simulink model "mbqpsk"  (R2019a)
settings: Solver=FixedStepDiscrete  StartTime=0.0  StopTime=inf  RelTol=1e-3  EnableMultiTasking=on
PreLoadFcn:
  | SimPars = simrfV2_qpsk_init();
  | load simrfV2_qpsk_patch_antenna.mat;
undefined symbols (not defined in the file or in its folder): lambda, P_isolated, phased, physconst
libraries: simrfV2util1 x44, simrfV2elements x40, simrfV2junction1 x28, simrfV2systems x8, commrflib2 x3, commdigbbndpm3 x3, dspsigops x3, dspmathops x3, phasedtxrxlib x3, commutil2 x2, commsequence2 x2, commsync2 x2
(part 1 of 2)
CloseFcn:
  | clear SimPars lambda P_isolated;
  | clear Spars;
Description:
  | Modeling an RF mmWave Transmitter with Hybrid Beamforming
settings Model: SimulationMode=accelerator  Creator=Arpan Samanta  LastModifiedBy=Arpan
settings DataIOCC: ExternalInput=txWaveform  InitialState=xFinal  SaveOperatingPoint=on  SaveFormat=Array  SaveOutput=off  SignalLogging=off  DSMLogging=off  SaveTime=off  ReturnWorkspaceOutputs=off  OutputSaveName=rx
settings OptimizationCC: DefaultParameterBehavior=Inlined  InlineInvariantSignals=on  EfficientMapNaN2IntZero=off  LifeSpan=inf  SimCompilerOptimization=on
settings DebuggingCC: ReadBeforeWriteMsg=DisableAll  WriteAfterWriteMsg=DisableAll  WriteAfterReadMsg=DisableAll  UnderspecifiedInitializationDetection=Classic  MergeDetectMultiDrivingBlocksExec=none  SolverPrmCheckMsg=warning  InheritedTsInSrcMsg=none  MultiTaskDSMMsg=none  IntegerOverflowMsg=none  AllowSymbolicDim=off  SFUnexpectedBacktrackingDiag=warning  SFNoUnconditionalDefaultTransitionDiag=none  SFUndirectedBroadcastEventsDiag=none  SFExecutionAtInitializationDiag=none  IntegerSaturationMsg=none  ArithmeticOperatorsInVariantConditions=warning
settings HardwareCC: ProdBitPerPointer=32  ProdBitPerSizeT=32  ProdBitPerPtrDiffT=32  ProdLargestAtomicFloat=None  ProdIntDivRoundTo=Undefined  ProdEndianess=Unspecified  ProdWordSize=32  ProdHWDeviceType=32-bit Generic  TargetBitPerPointer=64  TargetBitPerSizeT=64  TargetBitPerPtrDiffT=64  TargetLongLongMode=on  TargetIntDivRoundTo=Zero  TargetEndianess=LittleEndian  TargetWordSize=64  TargetHWDeviceType=MATLAB Host  ProdEqTarget=off
settings ModelReferenceCC: EnableParallelModelReferenceBuilds=on  PropagateSignalLabelsOutOfModel=off
settings SFSimCC: SFSimEcho=off  SimUseLocalCustomCode=off
settings RTWCC: RTWUseLocalCustomCode=off  BuildConfiguration=Faster Runs
settings CodeAppCC: MaxIdLength=128  StateflowObjectComments=on
settings GRTTargetCC: TargetLangStandard=C89/C90 (ANSI)  CombineOutputUpdateFcns=off  GRTInterface=on
settings ConfigComp: CovMetricSettings=dw  CovHtmlReporting=on  CovSaveCumulativeToWorkspaceVar=on  CovSaveSingleToWorkspaceVar=on  CovExternalEMLEnable=off  CovSFcnEnable=off
settings SimscapeCC: ExplicitSolverDiagnosticOptions=none  SimscapeNormalizeSystem=off

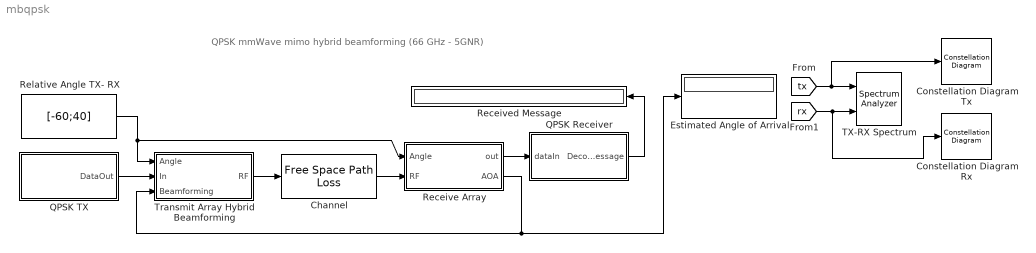
== system mbqpsk ==
  note: QPSK mmWave mimo hybrid beamforming (66 GHz - 5GNR)
  Channel : commrflib2/Free Space Path Loss  mode=Decibels  dB=50  d=0.100  fc=1920
      settings: SourceProductName=Communications Toolbox  SourceProductBaseCode=CM
  Constellation Diagram Rx : ConstellationDiagram
  Constellation Diagram Tx : ConstellationDiagram
  Estimated Angle of Arrival : Display
  QPSK Receiver : Subsystem
      mask Display: disp('QPSK \n Receiver');
  QPSK TX : Subsystem  mask{Power=-30}
      mask prompts: Power "Power (dBFS)"
      mask Display: disp('QPSK \n Transmitter')
  Receive Array : Subsystem
  Received Message : Display
  Relative Angle TX- RX : Constant  Value=[-60;40]  VectorParams1D=off
  TX-RX Spectrum : SpectrumAnalyzer  NumInputPorts=2
  Transmit Array Hybrid Beamforming : Subsystem
  wires:
  Channel/1 -> Receive Array/2(RF)
  Receive Array/1(out) -> QPSK Receiver/1(dataIn)
  Relative Angle TX- RX/1 -> Transmit Array Hybrid Beamforming/1(Angle), Receive Array/1(Angle)
  [tx] -> TX-RX Spectrum/1, Constellation Diagram Tx/1
  [rx] -> TX-RX Spectrum/2, Constellation Diagram Rx/1
  QPSK Receiver/1(Decoded Message) -> Received Message/1
  QPSK TX/1(DataOut) -> Transmit Array Hybrid Beamforming/2(In)
  Transmit Array Hybrid Beamforming/1(RF) -> Channel/1
  Receive Array/2(AOA) -> Estimated Angle of Arrival/1, Transmit Array Hybrid Beamforming/3(Beamforming)

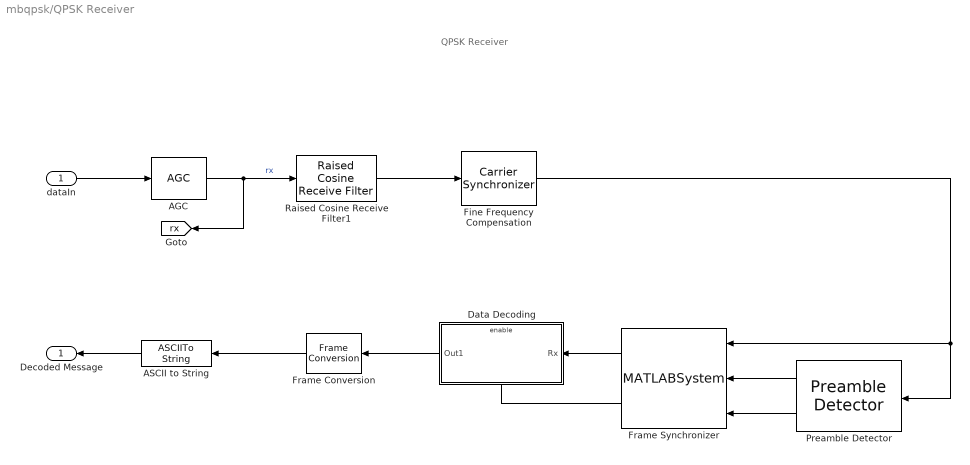
== system mbqpsk/QPSK Receiver ==
  note: QPSK Receiver
  dataIn : Inport
  AGC : commrfcorlib/AGC  LegacyMode=off  DetectorMethod=Rectifier  LoopMethod=Linear  UpdatePeriod=100  StepSize=0.1  AdaptationStepSize=0.01  DesiredOutputPower=1  AveragingLength=200  MaximumGain=30  MaxPowerGain=60  GainOutputPort=off  InputPowerOutputPort=off  SimulateUsing=Code generation
      settings: SourceProductName=Communications Toolbox
  ASCII to String : ASCIIToString
  Data Decoding : Subsystem
      mask Display: disp('Data Decoding');
  Fine Frequency Compensation : commsync2/Carrier Synchronizer  Modulation=QPSK  ModulationPhaseOffset=Auto  CustomPhaseOffset=0  SamplesPerSymbol=1  DampingFactor=1/sqrt(2)  NormalizedLoopBandwidth=0.005  EstimatedPhaseErrorOutputPort=off  SimulateUsing=Code generation
      settings: SourceProductName=Communications Toolbox
  Frame Conversion : FrameConversion  OutFrame=Sample-based
  Frame Synchronizer : MATLABSystem  System=comm.internal.examples.FrameSynchronizer  Input=Symbol  OutputFrameLength=SimPars.NumSymsPerFrame  PreambleLength=SimPars.BarkerLength  SimulateUsing=Code generation
      mask Type: comm.internal.examples.FrameSynchronizer
      mask Display:
      | disp(['Frame' char(10) 'Synchronizer']);
      | port_label('input',1,'u');
      | port_label('input',2,'idx');
      | port_label('input',3,'dtMt');
      | port_label('output',1,'Frame');
      | port_label('output',2,'Valid');
  Preamble Detector : commsync2/Preamble Detector  Input=Symbol  Preamble=sqrt(2)/2 * (-1-1i) *SimPars.BarkerCode  Threshold=10  DetectionMetricOutput=on  Detections=All  SimulateUsing=Code generation
      settings: SourceProductName=Communications Toolbox  SourceProductBaseCode=CM
  Raised Cosine Receive Filter1 : commfilt2/Raised Cosine Receive Filter  filtType=Square root  R=SimPars.RolloffFactor  filtSpan=SimPars.RCFilterSpan  N=SimPars.SamplesPerSymbol  downFactor=SimPars.RxRCFilterDecimation  downOffset=0  filterGain=1  InputProcessing=Columns as channels (frame based)  RateOptions=Enforce single-rate processing  framing=Mute  checkCoeff=off  variableName=rcRxFilt1  currentFiltSpan=10  D=5  inputOffset=0  sampMode=Mute  saveAsFlag=0  rateMode=Downsampling  checkGain=Normalized  launchFVT=on  roundingMode=Floor  overflowMode=off  coeffDataTypeStr=Inherit: Same word length as input  coeffMin=[]  coeffMax=[]  coeffLastDataTypeStr=Inherit: Same word length as input  accumDataTypeStr=Inherit: Same as product output  accumLastDataTypeStr=Inherit: Same as product output  outputDataTypeStr=Inherit: Same as accumulator  outputMin=[]  outputMax=[]  outputLastDataTypeStr=Inherit: Same as accumulator
      settings: SourceProductName=Communications Toolbox
  Decoded Message : Outport
  tag scope: rx=global
  wires:
  ASCII to String/1 -> Decoded Message/1
  Frame Conversion/1 -> ASCII to String/1
  AGC/1 -> Raised Cosine Receive Filter1/1, [rx]  "rx"
  Preamble Detector/1 -> Frame Synchronizer/2
  Frame Synchronizer/2 -> Data Decoding/Enable
  Frame Synchronizer/1 -> Data Decoding/1(Rx)
  Preamble Detector/2 -> Frame Synchronizer/3
  Fine Frequency Compensation/1 -> Frame Synchronizer/1, Preamble Detector/1
  Data Decoding/1(Out1) -> Frame Conversion/1
  dataIn/1 -> AGC/1
  Raised Cosine Receive Filter1/1 -> Fine Frequency Compensation/1

== system mbqpsk/QPSK TX ==
  note: QPSK Transmitter
  Bit Generation : Subsystem
      mask Display: disp('Bits Generation')
  Gain : Gain  Gain=sqrt(2)
  QPSK Modulator Baseband : commdigbbndpm3/QPSK Modulator Baseband  InType=Bit  Enc=Gray  Ph=pi/4  outDtype=double  outWordLen=16  outUDDataType=sfix(16)  outFracLenMode=Best precision  outFracLen=15  outDataTypeStr=double  outLastDataTypeStr=double
      settings: SourceProductName=Communications Toolbox
  Raised Cosine Transmit Filter1 : commfilt2/Raised Cosine Transmit Filter  filtType=Square root  R=SimPars.RolloffFactor  filtSpan=SimPars.RCFilterSpan  N=SimPars.SamplesPerSymbol  filterGain=1  InputProcessing=Columns as channels (frame based)  RateOptions=Enforce single-rate processing  framing=Mute  checkCoeff=off  variableName=rcTxFilt1  checkGain=Normalized  sampMode=Mute  saveAsFlag=0  currentFiltSpan=10  D=5  launchFVT=on  roundingMode=Floor  overflowMode=off  coeffDataTypeStr=Inherit: Same word length as input  coeffMin=[]  coeffMax=[]  coeffLastDataTypeStr=Inherit: Same word length as input  outputDataTypeStr=Inherit: Same as accumulator  outputMin=[]  outputMax=[]  outputLastDataTypeStr=Inherit: Same as accumulator
      settings: SourceProductName=Communications Toolbox
  Unbuffer : Unbuffer
  dB Gain : dspmathops/dB Gain  dB=Power-30+3  intype=Amplitude
      settings: SourceProductName=DSP System Toolbox  SourceProductBaseCode=DS
  DataOut : Outport
  tag scope: tx=global
  wires:
  Unbuffer/1 -> DataOut/1
  dB Gain/1 -> Unbuffer/1
  Bit Generation/1(Out) -> QPSK Modulator Baseband/1
  QPSK Modulator Baseband/1 -> Raised Cosine Transmit Filter1/1
  Raised Cosine Transmit Filter1/1 -> Gain/1, dB Gain/1
  Gain/1 -> [tx]  "tx"

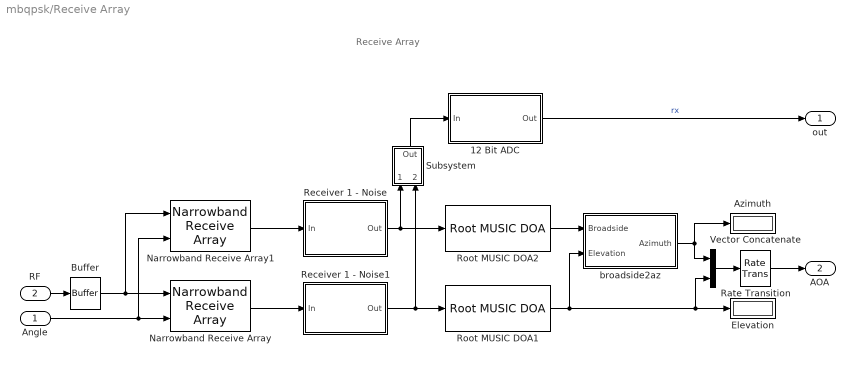
== system mbqpsk/Receive Array ==
  note: Receive Array
  Angle : Inport
  RF : Inport  Port=2
  12 Bit ADC : Subsystem  mask{FS_P_dBm=-10, N=12}
      mask prompts: FS_P_dBm "Full Scale Power (dBm)"
  Azimuth : Display
  Buffer : Buffer  N=SimPars.NumBitsPerFrame  OutputFrames=off
  Elevation : Display
  Narrowband Receive Array : phasedtxrxlib/Narrowband Receive Array  PropagationSpeed=physconst( 'LightSpeed' )  OperatingFrequency=SimPars.CarrierFreq  Wavefront=Plane  SensorGainMeasure=dB  Polarization=None  WeightsInputPort=off  SimulateUsing=Code generation  Sensor=phased.ULA('NumElements',4,'ElementSpacing',lambda/2,'ArrayAxis','z','Element',phased.IsotropicAntennaElement('BackBaffled',true))
      settings: SourceProductName=Phased Array System Toolbox  SourceProductBaseCode=AR
  Narrowband Receive Array1 : phasedtxrxlib/Narrowband Receive Array  PropagationSpeed=physconst( 'LightSpeed' )  OperatingFrequency=SimPars.CarrierFreq  Wavefront=Plane  SensorGainMeasure=dB  Polarization=None  WeightsInputPort=off  SimulateUsing=Code generation  Sensor=phased.ULA('NumElements',4,'ElementSpacing',lambda/2,'ArrayAxis','y','Element',phased.IsotropicAntennaElement('BackBaffled',true))
      settings: SourceProductName=Phased Array System Toolbox  SourceProductBaseCode=AR
  Rate Transition : RateTransition
  Receiver 1 - Noise : Subsystem  mask{NF=5, Gain=40, seed=123}
      mask prompts: NF "Noise Figure (dB)"; Gain "Gain (dB)"
      mask Display: disp('Receiver\n Gain/Noise')
  Receiver 1 - Noise1 : Subsystem  mask{NF=5, Gain=40, seed=3456}
      mask prompts: NF "Noise Figure (dB)"; Gain "Gain (dB)"
      mask Display: disp('Receiver\n Gain/Noise')
  Root MUSIC DOA1 : phaseddoalib/Root MUSIC DOA  PropagationSpeed=physconst( 'LightSpeed' )  OperatingFrequency=SimPars.CarrierFreq  NumSignalsSource=Property  NumSignalsMethod=AIC  NumSignals=1  ForwardBackwardAveraging=off  SpatialSmoothing=0  SimulateUsing=Code generation  SensorArray=phased.ULA('Element',phased.IsotropicAntennaElement('BackBaffled',true),'NumElements',4,'ElementSpacing',lambda/2,'ArrayAxis','z')
      settings: SourceProductName=Phased Array System Toolbox  SourceProductBaseCode=AR
  Root MUSIC DOA2 : phaseddoalib/Root MUSIC DOA  PropagationSpeed=physconst( 'LightSpeed' )  OperatingFrequency=SimPars.CarrierFreq  NumSignalsSource=Property  NumSignalsMethod=AIC  NumSignals=1  ForwardBackwardAveraging=off  SpatialSmoothing=0  SimulateUsing=Code generation  SensorArray=phased.ULA('Element',phased.IsotropicAntennaElement('BackBaffled',true),'NumElements',4,'ElementSpacing',0.5*lambda)
      settings: SourceProductName=Phased Array System Toolbox  SourceProductBaseCode=AR
  Subsystem : Subsystem
  Vector Concatenate : Concatenate  Mode=Multidimensional array
  broadside2az : Subsystem  VariantControl=BroadsideToAzimuth
  out : Outport
  AOA : Outport  Port=2
  wires:
  RF/1 -> Buffer/1
  broadside2az/1(Azimuth) -> Azimuth/1, Vector Concatenate/1
  Vector Concatenate/1 -> Rate Transition/1
  Angle/1 -> Narrowband Receive Array1/2, Narrowband Receive Array/2
  Root MUSIC DOA2/1 -> broadside2az/1(Broadside)
  Root MUSIC DOA1/1 -> Elevation/1, Vector Concatenate/2, broadside2az/2(Elevation)
  Narrowband Receive Array/1 -> Receiver 1 - Noise1/1(In)
  Narrowband Receive Array1/1 -> Receiver 1 - Noise/1(In)
  Receiver 1 - Noise/1(Out) -> Root MUSIC DOA2/1, Subsystem/1(In1)
  Receiver 1 - Noise1/1(Out) -> Root MUSIC DOA1/1, Subsystem/2(In2)
  Buffer/1 -> Narrowband Receive Array1/1, Narrowband Receive Array/1
  Rate Transition/1 -> AOA/1
  12 Bit ADC/1(Out) -> out/1  "rx"
  Subsystem/1(Out) -> 12 Bit ADC/1("In  ")

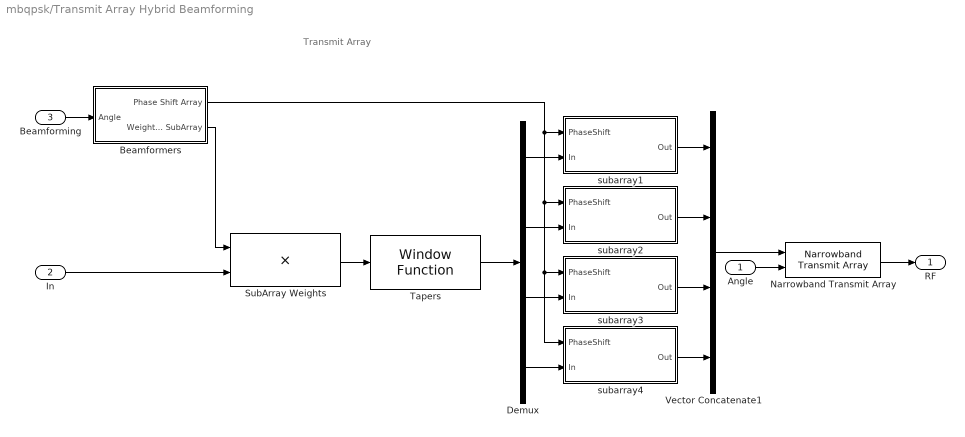
== system mbqpsk/Transmit Array Hybrid Beamforming ==
  note: Transmit Array
  Angle : Inport
  In : Inport  Port=2
  Beamforming : Inport  Port=3
  Beamformers : Subsystem
  Demux : Demux
  Narrowband Transmit Array : phasedtxrxlib/Narrowband Transmit Array  PropagationSpeed=physconst( 'LightSpeed' )  OperatingFrequency=SimPars.CarrierFreq  CombineRadiatedSignals=on  SensorGainMeasure=dB  Polarization=None  WeightsInputPort=off  SimulateUsing=Interpreted execution  Sensor=phased.URA('Size',[8, 4],'ElementSpacing',[0.5*lambda, 0.5*lambda],'Element',phased.CustomAntennaElement('AzimuthAngles',-180:5:180,'ElevationAngles',-90:5:90,'MagnitudePattern',P_isolated,'PhasePattern',zeros(37,73)))
      settings: SourceProductName=Phased Array System Toolbox  SourceProductBaseCode=AR
  SubArray Weights : Product
  Tapers : dspsigops/Window Function  winmode=Apply window to input  wintype=Hamming  sampmode=Continuous  samptime=1  N=64  Rs=50  beta=10  winsamp=Symmetric  UserWindow=hamming  OptParams=off  UserParams={'symmetric'}  dataType=double  isSigned=on  wordLen=16  udDataType=sfix(16)  fracBitsMode=Best precision  numFracBits=15  roundingMode=Floor  overflowMode=off  numSidelobes=4  sidelobeLevel=-30
      settings: SourceProductName=DSP System Toolbox  SourceProductBaseCode=DS
  Vector Concatenate1 : Concatenate  NumInputs=4  Mode=Multidimensional array  ConcatenateDimension=2
  subarray1 : Subsystem
  subarray2 : Subsystem
  subarray3 : Subsystem
  subarray4 : Subsystem
  RF : Outport
  wires:
  Demux/1 -> subarray1/2(In)
  Demux/2 -> subarray2/2(In)
  Demux/3 -> subarray3/2(In)
  Demux/4 -> subarray4/2(In)
  subarray1/1(Out) -> Vector Concatenate1/1
  subarray2/1(Out) -> Vector Concatenate1/2
  subarray3/1(Out) -> Vector Concatenate1/3
  subarray4/1(Out) -> Vector Concatenate1/4
  SubArray Weights/1 -> Tapers/1
  Beamformers/1(Phase Shift Array) -> subarray1/1(PhaseShift), subarray2/1(PhaseShift), subarray3/1(PhaseShift), subarray4/1(PhaseShift)
  Narrowband Transmit Array/1 -> RF/1
  Beamformers/2(Weights SubArray) -> SubArray Weights/1
  Beamforming/1 -> Beamformers/1(Angle)
  Vector Concatenate1/1 -> Narrowband Transmit Array/1
  In/1 -> SubArray Weights/2
  Angle/1 -> Narrowband Transmit Array/2
  Tapers/1 -> Demux/1

== system mbqpsk/QPSK Receiver/Data Decoding ==
  Rx : Inport
  Enable : EnablePort
  "Barker Code Symbol Generation " : Subsystem
      mask Display: disp('Barker Code\nSymbol Generation')
  Bit to Integer Converter : commutil2/Bit to Integer Converter  nbits=7  bitOrder=MSB first  signedOutputValues=Unsigned  outDtype=Inherit via internal rule  outDtypeSigned=Inherit via internal rule
      settings: SourceProductName=Communications Toolbox
  Descrambling : Subsystem
      mask Display: disp('Descrambling');
  Phase Ambiguity Correction & Demodulation : Subsystem
      mask Display: disp('Phase Ambiguity\nCorrection\n& Demodulation');
  Phase Offset Estimator : Subsystem
  Out1 : Outport
  wires:
  "Barker Code Symbol Generation "/1(Out) -> Phase Offset Estimator/1(BarkerRef)
  Phase Offset Estimator/1(Phase) -> Phase Ambiguity Correction & Demodulation/1(Phase)
  Rx/1 -> Phase Offset Estimator/2(Data), Phase Ambiguity Correction & Demodulation/2(Data)
  Descrambling/1(Out) -> Bit to Integer Converter/1
  Phase Ambiguity Correction & Demodulation/1(Out) -> Descrambling/1(In)
  Bit to Integer Converter/1 -> Out1/1

== system mbqpsk/QPSK TX/Bit Generation ==
  note: Each data frame contains 26 bits header (For Sync Purpose) and 174 data bits, first 105 data bits contain "Hello world ###" message. Scrambler is there to improve data transition density and frequency offset estimation.
  Barker Code SS : Subsystem
      mask Display: disp('Unipolar\nBarker Code')
  Matrix Concatenate : Concatenate  Mode=Multidimensional array
  Message Source : Subsystem
      mask Display: disp('Message\nSource')
  Repeat : dspsigops/Repeat  N=2  InputProcessing=Columns as channels (frame based)  RateOptions=Enforce single-rate processing  ic=0  mode=Unused parameter value
      settings: SourceProductName=DSP System Toolbox
  Scrambler : commsequence2/Scrambler  M=2  poly=[1 1 1 0 1]  iniStaSource=Dialog Parameter  ini_sta=[0 0 0 0]  resetViaPort=off
      settings: SourceProductName=Communications Toolbox  SourceProductBaseCode=CM
  Out : Outport
  wires:
  Barker Code SS/1(Out) -> Repeat/1
  Matrix Concatenate/1 -> Out/1
  Message Source/1(Out) -> Scrambler/1
  Repeat/1 -> Matrix Concatenate/1
  Scrambler/1 -> Matrix Concatenate/2

== system mbqpsk/Receive Array/12 Bit ADC ==
  "In  " : Inport
  Complex to Real-Imag : ComplexToRealImag
  Idealized ADC quantizer : simulink_extras/Additional Discrete/Idealized ADC quantizer  NumberOfConverterBits=N  Vmin=-10^((FS_P_dBm-30)/20)  Vmax=10^((FS_P_dBm-30)/20)  OutputDataType=double  OutputNegativeValues=on
      settings: SourceProductName=Simulink
  Idealized ADC quantizer1 : simulink_extras/Additional Discrete/Idealized ADC quantizer  NumberOfConverterBits=N  Vmin=-10^((FS_P_dBm-30)/20)  Vmax=10^((FS_P_dBm-30)/20)  OutputDataType=double  OutputNegativeValues=on
      settings: SourceProductName=Simulink
  Real-Imag to Complex : RealImagToComplex
  Out : Outport
  wires:
  "In  "/1 -> Complex to Real-Imag/1
  Complex to Real-Imag/1 -> Idealized ADC quantizer/1
  Complex to Real-Imag/2 -> Idealized ADC quantizer1/1
  Idealized ADC quantizer/1 -> Real-Imag to Complex/1
  Idealized ADC quantizer1/1 -> Real-Imag to Complex/2
  Real-Imag to Complex/1 -> Out/1

== system mbqpsk/Receive Array/Receiver 1 - Noise ==
  In : Inport
  Convert 1-D to 2-D : dspsigattribs/Convert 1-D to 2-D  M=200 % Frame  N=4  frameBasedOut=off
      settings: SourceProductName=DSP System Toolbox  SourceProductBaseCode=DS
  Receiver Thermal Noise : commrflib2/Receiver Thermal Noise  method=Noise figure  ntemp=290  nfigure=NF  nfactor=2  add290KAntennaNoise=on  seed=seed
      settings: SourceProductName=Communications Toolbox  SourceProductBaseCode=CM
  Reshape : Reshape  OutputDimensionality=Column vector (2-D)
  dB Gain : dspmathops/dB Gain  dB=Gain  intype=Amplitude
      settings: SourceProductName=DSP System Toolbox  SourceProductBaseCode=DS
  Out : Outport
  wires:
  In/1 -> Reshape/1
  Reshape/1 -> Receiver Thermal Noise/1
  Receiver Thermal Noise/1 -> dB Gain/1
  Convert 1-D to 2-D/1 -> Out/1
  dB Gain/1 -> Convert 1-D to 2-D/1

== system mbqpsk/Receive Array/Receiver 1 - Noise1 ==
  In : Inport
  Convert 1-D to 2-D : dspsigattribs/Convert 1-D to 2-D  M=200 % Frame  N=4  frameBasedOut=off
      settings: SourceProductName=DSP System Toolbox  SourceProductBaseCode=DS
  Receiver Thermal Noise : commrflib2/Receiver Thermal Noise  method=Noise figure  ntemp=290  nfigure=NF  nfactor=2  add290KAntennaNoise=on  seed=seed
      settings: SourceProductName=Communications Toolbox  SourceProductBaseCode=CM
  Reshape : Reshape  OutputDimensionality=Column vector (2-D)
  dB Gain : dspmathops/dB Gain  dB=Gain  intype=Amplitude
      settings: SourceProductName=DSP System Toolbox  SourceProductBaseCode=DS
  Out : Outport
  wires:
  dB Gain/1 -> Convert 1-D to 2-D/1
  Convert 1-D to 2-D/1 -> Out/1
  Receiver Thermal Noise/1 -> dB Gain/1
  Reshape/1 -> Receiver Thermal Noise/1
  In/1 -> Reshape/1

== system mbqpsk/Receive Array/Subsystem ==
  In1 : Inport
  In2 : Inport  Port=2
  Add : Sum
  Sum of Elements : Sum  Inputs=+  CollapseMode=Specified dimension  CollapseDim=2
  Sum of Elements1 : Sum  Inputs=+  CollapseMode=Specified dimension  CollapseDim=2
  Out : Outport
  wires:
  Sum of Elements/1 -> Add/1
  Sum of Elements1/1 -> Add/2
  Add/1 -> Out/1
  In2/1 -> Sum of Elements1/1
  In1/1 -> Sum of Elements/1

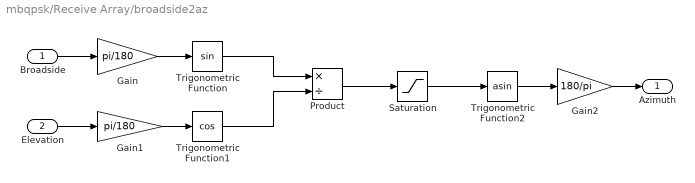
== system mbqpsk/Receive Array/broadside2az ==
  Broadside : Inport
  Elevation : Inport  Port=2
  Gain : Gain  Gain=pi/180
  Gain1 : Gain  Gain=pi/180
  Gain2 : Gain  Gain=180/pi
  Product : Product  Inputs=*/
  Saturation : Saturate  UpperLimit=1  LowerLimit=-1
  Trigonometric Function : Trigonometry
  Trigonometric Function1 : Trigonometry  Operator=cos
  Trigonometric Function2 : Trigonometry  Operator=asin
  Azimuth : Outport
  wires:
  Product/1 -> Saturation/1
  Gain2/1 -> Azimuth/1
  Trigonometric Function1/1 -> Product/2
  Trigonometric Function/1 -> Product/1
  Trigonometric Function2/1 -> Gain2/1
  Gain/1 -> Trigonometric Function/1
  Broadside/1 -> Gain/1
  Elevation/1 -> Gain1/1
  Gain1/1 -> Trigonometric Function1/1
  Saturation/1 -> Trigonometric Function2/1

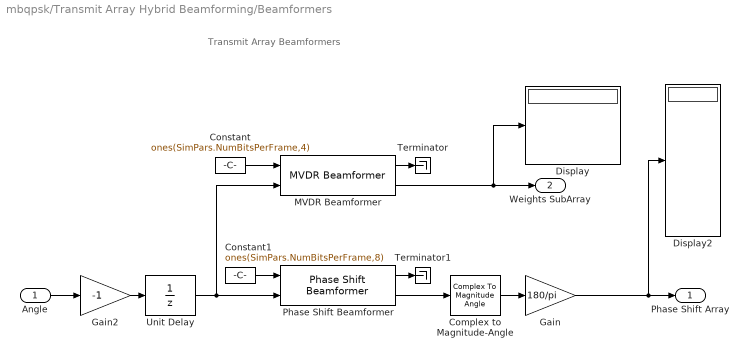
== system mbqpsk/Transmit Array Hybrid Beamforming/Beamformers ==
  note: Transmit Array Beamformers
  Angle : Inport
  Complex to Magnitude-Angle : ComplexToMagnitudeAngle  Output=Angle
  Constant : Constant  Value=ones(SimPars.NumBitsPerFrame,4)  VectorParams1D=off
  Constant1 : Constant  Value=ones(SimPars.NumBitsPerFrame,8)  VectorParams1D=off
  Display : Display
  Display2 : Display
  Gain : Gain  Gain=180/pi
  Gain2 : Gain  Gain=-1
  MVDR Beamformer : phasedbflib/MVDR Beamformer  PropagationSpeed=physconst( 'LightSpeed' )  OperatingFrequency=SimPars.CarrierFreq  DiagonalLoadingFactor=0.1  TrainingInputPort=off  DirectionSource=Input port  Direction=[ 0; 0 ]  NumPhaseShifterBits=0  WeightsOutputPort=on  SimulateUsing=Interpreted execution  SensorArray=phased.ReplicatedSubarray('GridSize',[ 1, 4],'GridSpacing',lambda/2,'SubarraySteering','Phase','PhaseShifterFrequency',SimPars.CarrierFreq,'Subarray',phased.ULA('NumElements',8,'ElementSpacing',lambda,'ArrayAxis','z','Element',phased.CustomAntennaElement('AzimuthAngles',-180:5:180,'ElevationAngles',-90:5:90,'MagnitudePattern',P_isolated,'PhasePattern',zeros(37,73))))
      settings: SourceProductName=Phased Array System Toolbox  SourceProductBaseCode=AR
  Phase Shift Beamformer : phasedbflib/Phase Shift Beamformer  PropagationSpeed=physconst( 'LightSpeed' )  OperatingFrequency=SimPars.CarrierFreq  DirectionSource=Input port  Direction=[ 0; 0 ]  NumPhaseShifterBits=0  WeightsNormalization=Distortionless  WeightsOutputPort=on  SimulateUsing=Interpreted execution  SensorArray=phased.ULA('Element',phased.CustomAntennaElement('AzimuthAngles',-180:5:180,'ElevationAngles',-90:5:90,'MagnitudePattern',P_isolated,'PhasePattern',zeros(37,73)),'NumElements',8,'ElementSpacing',0.5*lambda,'ArrayAxis','z')
      settings: SourceProductName=Phased Array System Toolbox  SourceProductBaseCode=AR
  Terminator : Terminator
  Terminator1 : Terminator
  Unit Delay : UnitDelay  SampleTime=-1  HasFrameUpgradeWarning=on
  Phase Shift Array : Outport
  Weights SubArray : Outport  Port=2
  wires:
  MVDR Beamformer/1 -> Terminator/1
  Complex to Magnitude-Angle/1 -> Gain/1
  Constant1/1 -> Phase Shift Beamformer/1
  Angle/1 -> Gain2/1
  Phase Shift Beamformer/1 -> Terminator1/1
  Constant/1 -> MVDR Beamformer/1
  Gain/1 -> Phase Shift Array/1, Display2/1
  Gain2/1 -> Unit Delay/1
  Unit Delay/1 -> MVDR Beamformer/2, Phase Shift Beamformer/2
  MVDR Beamformer/2 -> Weights SubArray/1, Display/1
  Phase Shift Beamformer/2 -> Complex to Magnitude-Angle/1

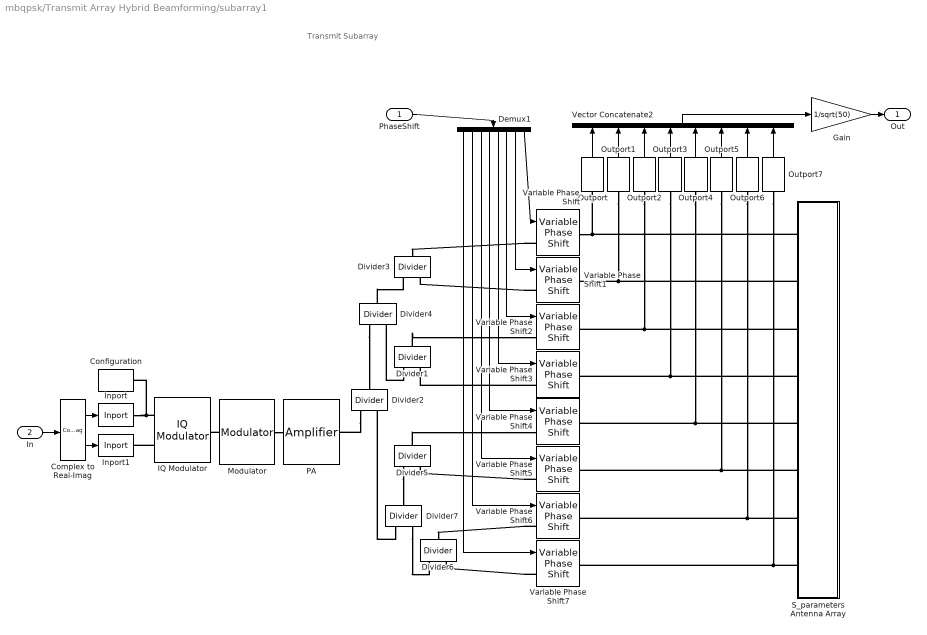
== system mbqpsk/Transmit Array Hybrid Beamforming/subarray1 ==
  note: Transmit Subarray
  PhaseShift : Inport  OutDataTypeStr=double  PortDimensions=[8 1]  SampleTime=[1.3020833333333334e-07,0]
  In : Inport  Port=2  OutDataTypeStr=double  PortDimensions=[1 1]  SampleTime=[1.3020833333333334e-07,0]
      settings: SignalType=complex
  Complex to Real-Imag : ComplexToRealImag
  Configuration : simrfV2util1/Configuration  AutoFreq=off  Tones="[5  66] GHz"  Harmonics=[3 1]  NormalizeCarrierPower=on  SolverType=Auto  UseCCode=on  StepSize=SimPars.SampleTime s  AddNoise=on  defaultRNG=on  Seed=0  Temperature=290.0 K  SolverDelFlag=0  AbsTol=1e-6  RelTol=1e-3  MaxIter=10  ErrorEstimationType=2-norm over all variables  EnableInterpFilter=off  HiddenFIRfilterControllerParam=off  SmallSignalApprox=off  AllSimFreqs=on  SimFreqs=[] Hz  SimFreqsInternal=[]
      settings: SourceProductName=RF Blockset  SourceProductBaseCode=RB
  Demux1 : Demux  Outputs=8
  Divider{1..7} (7 alike) : simrfV2junction1/Divider  classname=dividers  DataSource=Network-parameters  NumPorts=3  DeviceCirculator=Circulator clockwise  DeviceDivider=Wilkinson power divider  DeviceCoupler=Directional coupler  Paramtype=S-parameters  Sparam=[0 0 1; 1 0 0; 0 1 0]  SparamFreq=1e9 Hz  SparamZ0=50  Phase12=0  Phase33=0  Alpha=0  Coupling=0  Directivity=inf  InsertionLoss=inf  ReturnLoss=inf  InternalGrounding=on  SparamRepresentation=Frequency domain  FitOpt=Share all poles  FitTol=-40
      settings: SourceProductName=RF Blockset  SourceProductBaseCode=RB
  Gain : Gain  Gain=1/sqrt(50)
  IQ Modulator : simrfV2systems/IQ Modulator  classname=iqmod  Source_linear_gain=Available power gain  linear_gain=8 dB  Poly_Coeffs=[0 1]  LOFreq=5e9 Hz  Zin=50  Zout=50  AddIRFilters=off  AddCSFilter=off  InternalGrounding=on  ForceNextInit=off  NFloor=-168  GainMismatch=0.1 dB  PhaseMismatch=1.2 deg  Isolation=80 dB  AddPhaseNoise=off  PhaseNoiseOffset=1  PhaseNoiseLevel=-Inf  AutoImpulseLengthPN=on  ImpulseLengthPN=1e-10  ImpulseLength_unitPN=s  Source_Poly=Even and odd order  IPType=Output  IP2=21 dBm  IP3=30 dBm  P1dB=inf dBm  Psat=inf dBm  Gcomp=inf dBm  DesignMethodIR=Ideal  ResponseTypeIR=Lowpass  ImplementationIR=LC Tee  ImplementationIdealIR=Constant per carrier  UseFilterOrderIR=on  FilterOrderIR=3  PassFreq_lpIR=1  PassFreq_lp_unitIR=GHz  PassFreq_hpIR=2  PassFreq_hp_unitIR=GHz  PassFreq_bpIR=[2 3]  PassFreq_bp_unitIR=GHz  PassFreq_bsIR=[1 4]  PassFreq_bs_unitIR=GHz  PassAttenIR=10*log10(2)  StopFreq_lpIR=2  StopFreq_lp_unitIR=GHz  StopFreq_hpIR=1  StopFreq_hp_unitIR=GHz  StopFreq_bpIR=[1.5 3.5]  StopFreq_bp_unitIR=GHz  StopFreq_bsIR=[2.1 2.9]  StopFreq_bs_unitIR=GHz  StopAttenIR=40  RsrcIR=50  RloadIR=50  AutoImpulseLengthIR=on  ImpulseLengthIR=1e-10  ImpulseLength_unitIR=s  DesignMethodCS=Ideal  ResponseTypeCS=Highpass  ImplementationCS=LC Tee  ImplementationIdealCS=Constant per carrier  UseFilterOrderCS=on  FilterOrderCS=3  PassFreq_lpCS=1  PassFreq_lp_unitCS=GHz  PassFreq_hpCS=2  PassFreq_hp_unitCS=GHz  PassFreq_bpCS=[2 3]  PassFreq_bp_unitCS=GHz  PassFreq_bsCS=[1 4]  PassFreq_bs_unitCS=GHz  PassAttenCS=10*log10(2)  StopFreq_lpCS=2  StopFreq_lp_unitCS=GHz  StopFreq_hpCS=1  StopFreq_hp_unitCS=GHz  StopFreq_bpCS=[1.5 3.5]  StopFreq_bp_unitCS=GHz  StopFreq_bsCS=[2.1 2.9]  StopFreq_bs_unitCS=GHz  StopAttenCS=40  RsrcCS=50  RloadCS=50  AutoImpulseLengthCS=on  ImpulseLengthCS=1e-10  ImpulseLength_unitCS=s
      settings: SourceProductName=RF Blockset  SourceProductBaseCode=RB
  Inport : simrfV2util1/Inport  SimulinkInputSignalType=Power  CarrierFreq=0 Hz  ZS=50  InternalGrounding=on
      settings: SourceProductName=RF Blockset  SourceProductBaseCode=RB
  Inport1 : simrfV2util1/Inport  SimulinkInputSignalType=Power  CarrierFreq=0 Hz  ZS=50  InternalGrounding=on
      settings: SourceProductName=RF Blockset  SourceProductBaseCode=RB
  Modulator : simrfV2systems/Modulator  classname=rfmod  Source_linear_gain=Available power gain  linear_gain=-5 dB  Poly_Coeffs=[0 1]  LOFreq=61e9 Hz  Zin=50  Zout=50  AddIRFilter=on  AddCSFilter=on  InternalGrounding=on  ForceNextInit=off  Source_Poly=Even and odd order  IPType=Output  IP2=inf dBm  IP3=inf dBm  P1dB=inf dBm  Psat=inf dBm  Gcomp=inf dBm  NF=6  Isolation=100 dB  AddPhaseNoise=off  PhaseNoiseOffset=1  PhaseNoiseLevel=-Inf  AutoImpulseLengthPN=on  ImpulseLengthPN=1e-10  ImpulseLength_unitPN=s  DesignMethodIR=Ideal  ResponseTypeIR=Lowpass  ImplementationIR=LC Tee  ImplementationIdealIR=Constant per carrier  UseFilterOrderIR=on  FilterOrderIR=3  PassFreq_lpIR=10  PassFreq_lp_unitIR=GHz  PassFreq_hpIR=2  PassFreq_hp_unitIR=GHz  PassFreq_bpIR=[2 3]  PassFreq_bp_unitIR=GHz  PassFreq_bsIR=[1 4]  PassFreq_bs_unitIR=GHz  PassAttenIR=10*log10(2)  StopFreq_lpIR=2  StopFreq_lp_unitIR=GHz  StopFreq_hpIR=1  StopFreq_hp_unitIR=GHz  StopFreq_bpIR=[1.5 3.5]  StopFreq_bp_unitIR=GHz  StopFreq_bsIR=[2.1 2.9]  StopFreq_bs_unitIR=GHz  StopAttenIR=40  RsrcIR=50  RloadIR=50  AutoImpulseLengthIR=on  ImpulseLengthIR=1e-10  ImpulseLength_unitIR=s  DesignMethodCS=Ideal  ResponseTypeCS=Highpass  ImplementationCS=LC Tee  ImplementationIdealCS=Constant per carrier  UseFilterOrderCS=on  FilterOrderCS=3  PassFreq_lpCS=1  PassFreq_lp_unitCS=GHz  PassFreq_hpCS=60  PassFreq_hp_unitCS=GHz  PassFreq_bpCS=[2 3]  PassFreq_bp_unitCS=GHz  PassFreq_bsCS=[1 4]  PassFreq_bs_unitCS=GHz  PassAttenCS=10*log10(2)  StopFreq_lpCS=2  StopFreq_lp_unitCS=GHz  StopFreq_hpCS=1  StopFreq_hp_unitCS=GHz  StopFreq_bpCS=[1.5 3.5]  StopFreq_bp_unitCS=GHz  StopFreq_bsCS=[2.1 2.9]  StopFreq_bs_unitCS=GHz  StopAttenCS=40  RsrcCS=50  RloadCS=50  AutoImpulseLengthCS=on  ImpulseLengthCS=1e-10  ImpulseLength_unitCS=s
      settings: SourceProductName=RF Blockset  SourceProductBaseCode=RB
  Outport{,1..7} (8 alike) : simrfV2util1/Outport  SensorType=Ideal voltage  OutputFormat=Complex Baseband  CarrierFreq=SimPars.CarrierFreq Hz  ZL=Inf  InternalGrounding=on  StepSize=1e-6 s  AutoStep=on
      settings: SourceProductName=RF Blockset  SourceProductBaseCode=RB
  PA : simrfV2elements/Amplifier  classname=amplifier  DataSource=Data file  File=unitygain.s2p  Paramtype=S-parameters  Sparam=[0 0;1 0]  SparamFreq=1e9 Hz  SparamZ0=50  Residues=0  Poles=0  DF={0 0; 1 0}  Source_linear_gain=Available power gain  linear_gain=12 dB  Zin=50  Zout=50  Source_Poly=Odd order  Poly_Coeffs=[0 1]  IPType=Output  IP2=inf dBm  IP3=20 dBm  P1dB=33 dBm  Psat=inf dBm  Gcomp=inf dBm  InternalGrounding=on  SourceFreq=Extracted from data source  PlotFreq=[1e9:1e6:3e9] Hz  PlotType=X-Y plane  YParam1=S11  YFormat1=Magnitude (decibels)  YParam2=None  YFormat2=Magnitude (decibels)  YOption=Linear  XOption=Linear  SparamRepresentation=Time domain (rationalfit)  FitTol=-40  FitOpt=Fit individually  AutoImpulseLength=on  ImpulseLength=1e-10 s  MagModeling=off  AddNoise=on  NoiseType=Noise figure  NoiseDist=White  NF=3  MinNF=0  Gopt=0  RN=0  CarrierFreq=0 Hz  NoiseAutoImpulseLength=on  NoiseImpulseLength=1e-10 s  SpecifyOpFreq=off  OpFreq=0 Hz
      settings: SourceProductName=RF Blockset  SourceProductBaseCode=RB
  S_parameters Antenna Array : Subsystem
  Variable Phase Shift{,1..7} (8 alike) : simrfV2elements/Variable Phase Shift  classname=varphase  PhaseShift_unit=deg  SparamZ0=50  InternalGrounding=on
      settings: SourceProductName=RF Blockset  SourceProductBaseCode=RB
  Vector Concatenate2 : Concatenate  NumInputs=8  Mode=Multidimensional array  ConcatenateDimension=2
  Out : Outport  OutDataTypeStr=double  PortDimensions=[1 8]  SampleTime=[1.3020833333333334e-07,0]
      settings: SignalType=complex
  wires:
  Outport1/1 -> Vector Concatenate2/2
  Demux1/1 -> Variable Phase Shift7/1
  Demux1/8 -> Variable Phase Shift/1
  Outport6/1 -> Vector Concatenate2/7
  Outport4/1 -> Vector Concatenate2/5
  Complex to Real-Imag/2 -> Inport1/1
  Demux1/7 -> Variable Phase Shift1/1
  Demux1/6 -> Variable Phase Shift2/1
  Demux1/5 -> Variable Phase Shift3/1
  Outport/1 -> Vector Concatenate2/1
  In/1 -> Complex to Real-Imag/1
  Vector Concatenate2/1 -> Gain/1
  Complex to Real-Imag/1 -> Inport/1
  Outport2/1 -> Vector Concatenate2/3
  PhaseShift/1 -> Demux1/1
  Outport5/1 -> Vector Concatenate2/6
  Outport3/1 -> Vector Concatenate2/4
  Demux1/2 -> Variable Phase Shift6/1
  Demux1/3 -> Variable Phase Shift5/1
  Outport7/1 -> Vector Concatenate2/8
  Demux1/4 -> Variable Phase Shift4/1
  Gain/1 -> Out/1
  connections:
  Variable Phase Shift/LConn1 -- Divider3/RConn1
  Outport1/LConn1 -- S_parameters Antenna Array/RConn2 -- Variable Phase Shift1/RConn1
  Divider2/LConn1 -- PA/RConn1
  Outport3/LConn1 -- S_parameters Antenna Array/RConn4 -- Variable Phase Shift3/RConn1
  IQ Modulator/LConn2 -- Inport1/RConn1
  Outport7/LConn1 -- S_parameters Antenna Array/RConn8 -- Variable Phase Shift7/RConn1
  Variable Phase Shift7/LConn1 -- Divider6/LConn2
  Inport/RConn1 -- IQ Modulator/LConn1 -- Configuration/LConn1
  Variable Phase Shift3/LConn1 -- Divider1/LConn2
  Variable Phase Shift/RConn1 -- S_parameters Antenna Array/RConn1 -- Outport/LConn1
  Modulator/RConn1 -- PA/LConn1
  Outport2/LConn1 -- S_parameters Antenna Array/RConn3 -- Variable Phase Shift2/RConn1
  Variable Phase Shift5/LConn1 -- Divider5/LConn2
  Outport6/LConn1 -- S_parameters Antenna Array/RConn7 -- Variable Phase Shift6/RConn1
  Outport5/LConn1 -- S_parameters Antenna Array/RConn6 -- Variable Phase Shift5/RConn1
  Variable Phase Shift6/LConn1 -- Divider6/RConn1
  Divider5/RConn1 -- Variable Phase Shift4/LConn1
  Divider1/RConn1 -- Variable Phase Shift2/LConn1
  Divider4/LConn1 -- Divider2/RConn1
  Divider4/RConn1 -- Divider3/LConn1
  Divider1/LConn1 -- Divider4/LConn2
  Divider5/LConn1 -- Divider7/RConn1
  Divider7/LConn2 -- Divider6/LConn1
  Divider7/LConn1 -- Divider2/LConn2
  Variable Phase Shift1/LConn1 -- Divider3/LConn2
  Modulator/LConn1 -- IQ Modulator/RConn1
  Outport4/LConn1 -- S_parameters Antenna Array/RConn5 -- Variable Phase Shift4/RConn1

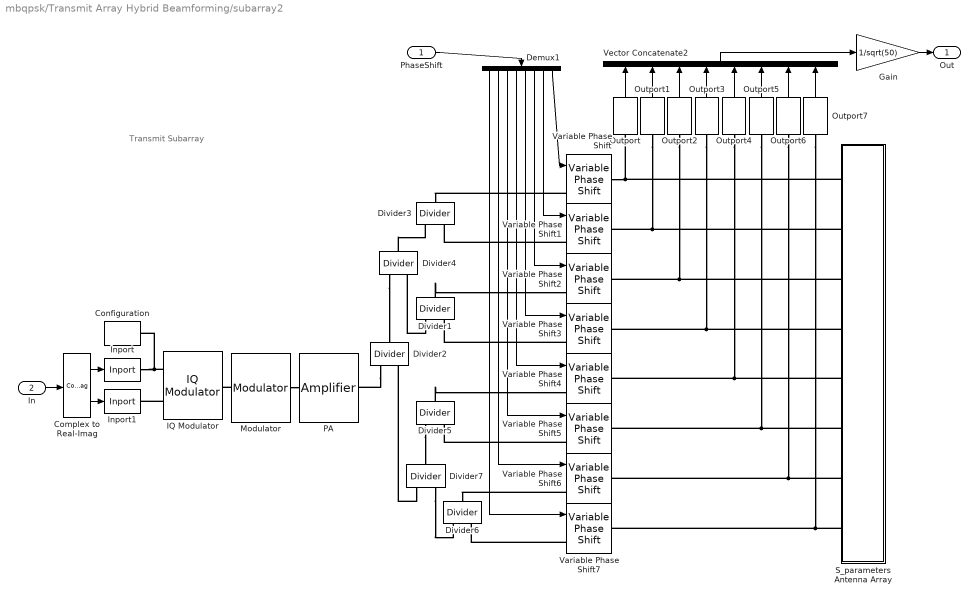
== system mbqpsk/Transmit Array Hybrid Beamforming/subarray2 ==
  note: Transmit Subarray
  PhaseShift : Inport  OutDataTypeStr=double  PortDimensions=[8 1]  SampleTime=[1.3020833333333334e-07,0]
  In : Inport  Port=2  OutDataTypeStr=double  PortDimensions=[1 1]  SampleTime=[1.3020833333333334e-07,0]
      settings: SignalType=complex
  Complex to Real-Imag : ComplexToRealImag
  Configuration : simrfV2util1/Configuration  AutoFreq=off  Tones="[5  66] GHz"  Harmonics=[3 1]  NormalizeCarrierPower=on  SolverType=Auto  UseCCode=on  StepSize=SimPars.SampleTime s  AddNoise=on  defaultRNG=on  Seed=0  Temperature=290.0 K  SolverDelFlag=0  AbsTol=1e-6  RelTol=1e-3  MaxIter=10  ErrorEstimationType=2-norm over all variables  EnableInterpFilter=off  HiddenFIRfilterControllerParam=off  SmallSignalApprox=off  AllSimFreqs=on  SimFreqs=[] Hz  SimFreqsInternal=[]
      settings: SourceProductName=RF Blockset  SourceProductBaseCode=RB
  Demux1 : Demux  Outputs=8
  Divider{1..7} (7 alike) : simrfV2junction1/Divider  classname=dividers  DataSource=Network-parameters  NumPorts=3  DeviceCirculator=Circulator clockwise  DeviceDivider=Wilkinson power divider  DeviceCoupler=Directional coupler  Paramtype=S-parameters  Sparam=[0 0 1; 1 0 0; 0 1 0]  SparamFreq=1e9 Hz  SparamZ0=50  Phase12=0  Phase33=0  Alpha=0  Coupling=0  Directivity=inf  InsertionLoss=inf  ReturnLoss=inf  InternalGrounding=on  SparamRepresentation=Frequency domain  FitOpt=Share all poles  FitTol=-40
      settings: SourceProductName=RF Blockset  SourceProductBaseCode=RB
  Gain : Gain  Gain=1/sqrt(50)
  IQ Modulator : simrfV2systems/IQ Modulator  classname=iqmod  Source_linear_gain=Available power gain  linear_gain=8 dB  Poly_Coeffs=[0 1]  LOFreq=5e9 Hz  Zin=50  Zout=50  AddIRFilters=off  AddCSFilter=off  InternalGrounding=on  ForceNextInit=off  NFloor=-168  GainMismatch=0.1 dB  PhaseMismatch=1.2 deg  Isolation=80 dB  AddPhaseNoise=off  PhaseNoiseOffset=1  PhaseNoiseLevel=-Inf  AutoImpulseLengthPN=on  ImpulseLengthPN=1e-10  ImpulseLength_unitPN=s  Source_Poly=Even and odd order  IPType=Output  IP2=21 dBm  IP3=30 dBm  P1dB=inf dBm  Psat=inf dBm  Gcomp=inf dBm  DesignMethodIR=Ideal  ResponseTypeIR=Lowpass  ImplementationIR=LC Tee  ImplementationIdealIR=Constant per carrier  UseFilterOrderIR=on  FilterOrderIR=3  PassFreq_lpIR=1  PassFreq_lp_unitIR=GHz  PassFreq_hpIR=2  PassFreq_hp_unitIR=GHz  PassFreq_bpIR=[2 3]  PassFreq_bp_unitIR=GHz  PassFreq_bsIR=[1 4]  PassFreq_bs_unitIR=GHz  PassAttenIR=10*log10(2)  StopFreq_lpIR=2  StopFreq_lp_unitIR=GHz  StopFreq_hpIR=1  StopFreq_hp_unitIR=GHz  StopFreq_bpIR=[1.5 3.5]  StopFreq_bp_unitIR=GHz  StopFreq_bsIR=[2.1 2.9]  StopFreq_bs_unitIR=GHz  StopAttenIR=40  RsrcIR=50  RloadIR=50  AutoImpulseLengthIR=on  ImpulseLengthIR=1e-10  ImpulseLength_unitIR=s  DesignMethodCS=Ideal  ResponseTypeCS=Highpass  ImplementationCS=LC Tee  ImplementationIdealCS=Constant per carrier  UseFilterOrderCS=on  FilterOrderCS=3  PassFreq_lpCS=1  PassFreq_lp_unitCS=GHz  PassFreq_hpCS=2  PassFreq_hp_unitCS=GHz  PassFreq_bpCS=[2 3]  PassFreq_bp_unitCS=GHz  PassFreq_bsCS=[1 4]  PassFreq_bs_unitCS=GHz  PassAttenCS=10*log10(2)  StopFreq_lpCS=2  StopFreq_lp_unitCS=GHz  StopFreq_hpCS=1  StopFreq_hp_unitCS=GHz  StopFreq_bpCS=[1.5 3.5]  StopFreq_bp_unitCS=GHz  StopFreq_bsCS=[2.1 2.9]  StopFreq_bs_unitCS=GHz  StopAttenCS=40  RsrcCS=50  RloadCS=50  AutoImpulseLengthCS=on  ImpulseLengthCS=1e-10  ImpulseLength_unitCS=s
      settings: SourceProductName=RF Blockset  SourceProductBaseCode=RB
  Inport : simrfV2util1/Inport  SimulinkInputSignalType=Power  CarrierFreq=0 Hz  ZS=50  InternalGrounding=on
      settings: SourceProductName=RF Blockset  SourceProductBaseCode=RB
  Inport1 : simrfV2util1/Inport  SimulinkInputSignalType=Power  CarrierFreq=0 Hz  ZS=50  InternalGrounding=on
      settings: SourceProductName=RF Blockset  SourceProductBaseCode=RB
  Modulator : simrfV2systems/Modulator  classname=rfmod  Source_linear_gain=Available power gain  linear_gain=-5 dB  Poly_Coeffs=[0 1]  LOFreq=61e9 Hz  Zin=50  Zout=50  AddIRFilter=on  AddCSFilter=on  InternalGrounding=on  ForceNextInit=off  Source_Poly=Even and odd order  IPType=Output  IP2=inf dBm  IP3=inf dBm  P1dB=inf dBm  Psat=inf dBm  Gcomp=inf dBm  NF=6  Isolation=100 dB  AddPhaseNoise=off  PhaseNoiseOffset=1  PhaseNoiseLevel=-Inf  AutoImpulseLengthPN=on  ImpulseLengthPN=1e-10  ImpulseLength_unitPN=s  DesignMethodIR=Ideal  ResponseTypeIR=Lowpass  ImplementationIR=LC Tee  ImplementationIdealIR=Constant per carrier  UseFilterOrderIR=on  FilterOrderIR=3  PassFreq_lpIR=10  PassFreq_lp_unitIR=GHz  PassFreq_hpIR=2  PassFreq_hp_unitIR=GHz  PassFreq_bpIR=[2 3]  PassFreq_bp_unitIR=GHz  PassFreq_bsIR=[1 4]  PassFreq_bs_unitIR=GHz  PassAttenIR=10*log10(2)  StopFreq_lpIR=2  StopFreq_lp_unitIR=GHz  StopFreq_hpIR=1  StopFreq_hp_unitIR=GHz  StopFreq_bpIR=[1.5 3.5]  StopFreq_bp_unitIR=GHz  StopFreq_bsIR=[2.1 2.9]  StopFreq_bs_unitIR=GHz  StopAttenIR=40  RsrcIR=50  RloadIR=50  AutoImpulseLengthIR=on  ImpulseLengthIR=1e-10  ImpulseLength_unitIR=s  DesignMethodCS=Ideal  ResponseTypeCS=Highpass  ImplementationCS=LC Tee  ImplementationIdealCS=Constant per carrier  UseFilterOrderCS=on  FilterOrderCS=3  PassFreq_lpCS=1  PassFreq_lp_unitCS=GHz  PassFreq_hpCS=60  PassFreq_hp_unitCS=GHz  PassFreq_bpCS=[2 3]  PassFreq_bp_unitCS=GHz  PassFreq_bsCS=[1 4]  PassFreq_bs_unitCS=GHz  PassAttenCS=10*log10(2)  StopFreq_lpCS=2  StopFreq_lp_unitCS=GHz  StopFreq_hpCS=1  StopFreq_hp_unitCS=GHz  StopFreq_bpCS=[1.5 3.5]  StopFreq_bp_unitCS=GHz  StopFreq_bsCS=[2.1 2.9]  StopFreq_bs_unitCS=GHz  StopAttenCS=40  RsrcCS=50  RloadCS=50  AutoImpulseLengthCS=on  ImpulseLengthCS=1e-10  ImpulseLength_unitCS=s
      settings: SourceProductName=RF Blockset  SourceProductBaseCode=RB
  Outport{,1..7} (8 alike) : simrfV2util1/Outport  SensorType=Ideal voltage  OutputFormat=Complex Baseband  CarrierFreq=SimPars.CarrierFreq Hz  ZL=Inf  InternalGrounding=on  StepSize=1e-6 s  AutoStep=on
      settings: SourceProductName=RF Blockset  SourceProductBaseCode=RB
  PA : simrfV2elements/Amplifier  classname=amplifier  DataSource=Data file  File=unitygain.s2p  Paramtype=S-parameters  Sparam=[0 0;1 0]  SparamFreq=1e9 Hz  SparamZ0=50  Residues=0  Poles=0  DF={0 0; 1 0}  Source_linear_gain=Available power gain  linear_gain=12 dB  Zin=50  Zout=50  Source_Poly=Odd order  Poly_Coeffs=[0 1]  IPType=Output  IP2=inf dBm  IP3=20 dBm  P1dB=33 dBm  Psat=inf dBm  Gcomp=inf dBm  InternalGrounding=on  SourceFreq=Extracted from data source  PlotFreq=[1e9:1e6:3e9] Hz  PlotType=X-Y plane  YParam1=S11  YFormat1=Magnitude (decibels)  YParam2=None  YFormat2=Magnitude (decibels)  YOption=Linear  XOption=Linear  SparamRepresentation=Time domain (rationalfit)  FitTol=-40  FitOpt=Fit individually  AutoImpulseLength=on  ImpulseLength=1e-10 s  MagModeling=off  AddNoise=on  NoiseType=Noise figure  NoiseDist=White  NF=3  MinNF=0  Gopt=0  RN=0  CarrierFreq=0 Hz  NoiseAutoImpulseLength=on  NoiseImpulseLength=1e-10 s  SpecifyOpFreq=off  OpFreq=0 Hz
      settings: SourceProductName=RF Blockset  SourceProductBaseCode=RB
  S_parameters Antenna Array : Subsystem
  Variable Phase Shift{,1..7} (8 alike) : simrfV2elements/Variable Phase Shift  classname=varphase  PhaseShift_unit=deg  SparamZ0=50  InternalGrounding=on
      settings: SourceProductName=RF Blockset  SourceProductBaseCode=RB
  Vector Concatenate2 : Concatenate  NumInputs=8  Mode=Multidimensional array  ConcatenateDimension=2
  Out : Outport  OutDataTypeStr=double  PortDimensions=[1 8]  SampleTime=[1.3020833333333334e-07,0]
      settings: SignalType=complex
  wires:
  Outport1/1 -> Vector Concatenate2/2
  Demux1/1 -> Variable Phase Shift7/1
  Demux1/8 -> Variable Phase Shift/1
  Outport6/1 -> Vector Concatenate2/7
  Outport4/1 -> Vector Concatenate2/5
  Complex to Real-Imag/2 -> Inport1/1
  Demux1/7 -> Variable Phase Shift1/1
  Demux1/6 -> Variable Phase Shift2/1
  Demux1/5 -> Variable Phase Shift3/1
  Outport/1 -> Vector Concatenate2/1
  In/1 -> Complex to Real-Imag/1
  Vector Concatenate2/1 -> Gain/1
  Complex to Real-Imag/1 -> Inport/1
  Outport2/1 -> Vector Concatenate2/3
  PhaseShift/1 -> Demux1/1
  Outport5/1 -> Vector Concatenate2/6
  Outport3/1 -> Vector Concatenate2/4
  Demux1/2 -> Variable Phase Shift6/1
  Demux1/3 -> Variable Phase Shift5/1
  Outport7/1 -> Vector Concatenate2/8
  Demux1/4 -> Variable Phase Shift4/1
  Gain/1 -> Out/1
  connections:
  Variable Phase Shift/LConn1 -- Divider3/RConn1
  Outport1/LConn1 -- S_parameters Antenna Array/RConn2 -- Variable Phase Shift1/RConn1
  Divider2/LConn1 -- PA/RConn1
  Outport3/LConn1 -- S_parameters Antenna Array/RConn4 -- Variable Phase Shift3/RConn1
  IQ Modulator/LConn2 -- Inport1/RConn1
  Outport7/LConn1 -- S_parameters Antenna Array/RConn8 -- Variable Phase Shift7/RConn1
  Variable Phase Shift7/LConn1 -- Divider6/LConn2
  Inport/RConn1 -- IQ Modulator/LConn1 -- Configuration/LConn1
  Variable Phase Shift3/LConn1 -- Divider1/LConn2
  Variable Phase Shift/RConn1 -- Outport/LConn1 -- S_parameters Antenna Array/RConn1
  Modulator/RConn1 -- PA/LConn1
  Outport2/LConn1 -- S_parameters Antenna Array/RConn3 -- Variable Phase Shift2/RConn1
  Variable Phase Shift5/LConn1 -- Divider5/LConn2
  Outport6/LConn1 -- S_parameters Antenna Array/RConn7 -- Variable Phase Shift6/RConn1
  Outport5/LConn1 -- S_parameters Antenna Array/RConn6 -- Variable Phase Shift5/RConn1
  Variable Phase Shift6/LConn1 -- Divider6/RConn1
  Divider5/RConn1 -- Variable Phase Shift4/LConn1
  Divider1/RConn1 -- Variable Phase Shift2/LConn1
  Divider4/LConn1 -- Divider2/RConn1
  Divider4/RConn1 -- Divider3/LConn1
  Divider1/LConn1 -- Divider4/LConn2
  Divider5/LConn1 -- Divider7/RConn1
  Divider7/LConn2 -- Divider6/LConn1
  Divider7/LConn1 -- Divider2/LConn2
  Variable Phase Shift1/LConn1 -- Divider3/LConn2
  Modulator/LConn1 -- IQ Modulator/RConn1
  Outport4/LConn1 -- S_parameters Antenna Array/RConn5 -- Variable Phase Shift4/RConn1
